simulink model "pendulum"  (R2021a)
settings: Solver=VariableStepAuto  StartTime=0.0  StopTime=10.0  RelTol=1e-3
undefined symbols (not defined in the file or in its folder): magnitude
settings Model: Creator=davidrico  LastModifiedBy=davidrico

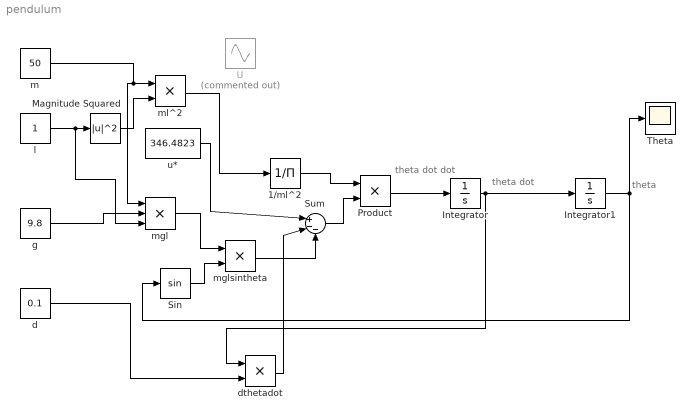
== system pendulum ==
  note: theta
  note: theta dot
  note: theta dot dot
  1/ml^2 : Product  Inputs=/
  Integrator : Integrator
  Integrator1 : Integrator
  Magnitude Squared : Math  Operator=magnitude^2  SaturateOnIntegerOverflow=on
  Product : Product
  Sin : Trigonometry
  Sum : Sum  Inputs=|+--
  Theta : Scope
  U : Sin  Commented=on  SampleTime=0
  d : Constant  Value=0.1
  dthetadot : Product
  g : Constant  Value=9.8
  l : Constant
  m : Constant  Value=50
  mgl : Product  Inputs=3
  mglsintheta : Product
  ml^2 : Product
  u* : Constant  Value=346.4823
  wires:
  l/1 -> mgl/3, Magnitude Squared/1
  m/1 -> mgl/1, ml^2/1
  Magnitude Squared/1 -> ml^2/2
  ml^2/1 -> 1/ml^2/1
  g/1 -> mgl/2
  1/ml^2/1 -> Product/1
  Product/1 -> Integrator/1
  Integrator/1 -> dthetadot/1, Integrator1/1
  Integrator1/1 -> Theta/1, Sin/1
  Sin/1 -> mglsintheta/2
  mgl/1 -> mglsintheta/1
  d/1 -> dthetadot/2
  dthetadot/1 -> Sum/2
  mglsintheta/1 -> Sum/3
  Sum/1 -> Product/2
  u*/1 -> Sum/1
